simulink model "rgb2grey_hw"  (R2019a)
settings: Solver=FixedStepDiscrete  StartTime=0.0  StopTime=inf  RelTol=1e-3
undefined symbols (not defined in the file): HDTV, Rec
libraries: visionzynq_privlib x3, dspvision x1, hdlsllib x1, visionsinks x1, visionzynqlib x1
settings Model: DataTypeOverride=Off  SimulationMode=accelerator  Creator=lbai  LastModifiedBy=lbai
settings DataIOCC: LimitDataPoints=on  SaveOutput=off  SignalLogging=off  DSMLogging=off  VisualizeSimOutput=off  SaveTime=off
settings OptimizationCC: BlockReduction=off  ConditionallyExecuteInputs=off  DefaultParameterBehavior=Inlined  LifeSpan=inf  SimCompilerOptimization=on
settings DebuggingCC: AlgebraicLoopMsg=error  SingleTaskRateTransMsg=error  ParameterPrecisionLossMsg=none  AllowSymbolicDim=off  PregeneratedLibrarySubsystemCodeDiagnostic=none  SFUnexpectedBacktrackingDiag=warning  SFNoUnconditionalDefaultTransitionDiag=warning  SFExecutionAtInitializationDiag=none  IntegerSaturationMsg=none  ArithmeticOperatorsInVariantConditions=warning
settings HardwareCC: ProdBitPerPointer=32  ProdBitPerSizeT=32  ProdBitPerPtrDiffT=32  ProdLargestAtomicFloat=None  ProdIntDivRoundTo=Undefined  ProdEndianess=Unspecified  ProdWordSize=32  ProdHWDeviceType=ASIC/FPGA->ASIC/FPGA  ProdEqTarget=off
settings SFSimCC: SimUseLocalCustomCode=off
settings RTWCC: RTWUseLocalCustomCode=off  BuildConfiguration=Faster Runs
settings CodeAppCC: StateflowObjectComments=on
settings GRTTargetCC: TargetLangStandard=C89/C90 (ANSI)  GeneratePreprocessorConditionals=Disable all
settings ConfigComp: CovMetricSettings=dw  CovHtmlReporting=on  CovSaveCumulativeToWorkspaceVar=on  CovSaveSingleToWorkspaceVar=on  CovExternalEMLEnable=off  CovSFcnEnable=off

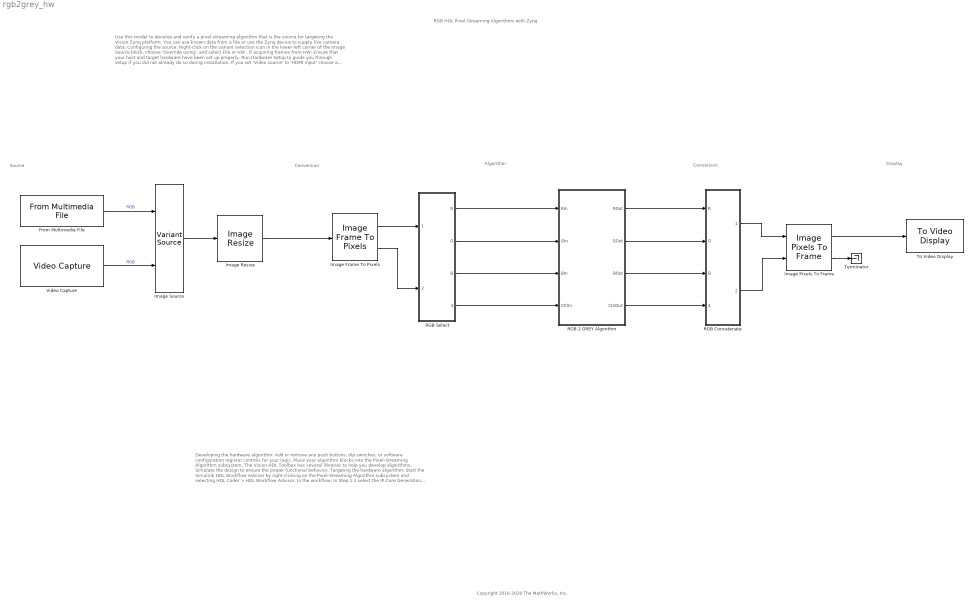
== system rgb2grey_hw ==
  note: Developing the hardware algorithm:
      | Add or remove any push buttons, dip switches, or software configuration register controls for your logic.
      | Place your algorithm blocks into the Pixel-Streaming Algorithm subsystem. The Vision HDL Toolbox has several libraries to help you develop algorithms.
      | Simulate the design to ensure the proper functional behavior.
      |
      | Targeting the hardware algorithm:
      |
      | Start the Simulink HDL Workflow Advisor by right-clicking on the Pixel-Streaming Algorithm subsystem and selecting HDL Coder > HDL Workflow Advisor.
      | In the workflow:
      | In Step 1.1 select the IP Core Generation workflow
      | In Step 1.1 select one of ZedBoard FMC-HDMI-CAM, ZC702 FMC-HDMI-CAM, ZC706 FMC-HDMI-CAM,
      | PicoZed FMC-HDMI-CAM.
      | In Step 1.2 select the reference platform that matches the desired pixel format.
      | In Step 1.3 map the reference design signals to the ports of the Pixel-Streaming Algorithm subsystem.
  note: Conversion
  note: Use this model to develop and verify a pixel-streaming algorithm that is the source for targeting the Vision Zynq platform. You can use known data from a file or use the Zynq device to supply live camera data.
      |
      | Configuring the source:
      | Right-click on the variant selection icon in the lower-left corner of the Image Source block, choose 'Override using', and select File or HW .
      | If acquiring frames from HW:
      | Ensure that your host and target hardware have been set up properly. Run Hardware Setup to guide you through setup if you did not already do so during installation.
      | If you set 'Video source' to 'HDMI input' choose a frame size that matches your camera settings.
      | If you set 'Video source' to 'Test pattern generator' choose any listed resolution. The hardware generates a color bar test pattern, and does not need an attached camera. It still requires the FMC board.
      | Since pixel-streaming algorithms will run many times slower than behavioral algorithms, consider adding a Resize block from Computer Vision System Toolbox to reduce the frame size that the algorithm operates on.
      |
      | Configuring conversions:
      | Ensure your Frame to Pixel and Pixel to Frame blocks match your source frame size.
  note: RGB HDL Pixel-Streaming Algorithms with Zynq
  note: Source
  note: Algorithm
  note: Display
  note: Conversion
  note: Copyright 2016-2018 The MathWorks, Inc.
  From Multimedia File : dspvision/From Multimedia File  inputFilename=vzSample1080p.avi  readRange=[1 Inf]  loop=on  numPlays=inf  outputStreams=Video only  videoDataType=uint8  audioDataType=int16  inheritSampleTime=off  userDefinedSampleTime=1/60  noAudioOutput=off  isIntensityVideo=off  fourcc=RGB  colorVideoFormat=One multidimensional signal  outputEOF=off  dataOrg=Column-major  audioFrameSize=1024  computeAudioFrameSize=off  outSamplingMode=Sample based
      settings: SourceProductName=DSP System Toolbox  SourceProductBaseCode=DS
  "Image Frame To Pixels " : visionzynq_privlib/Image Frame To Pixels   FrameSize=320x240p
      settings: SourceProductName=Computer Vision Toolbox Support Package for Xilinx Zynq-Based Hardware  SourceProductBaseCode=VP_VISION_ZYNQ
  Image Pixels To Frame : visionzynq_privlib/Image Pixels To Frame  FrameSize=320x240p
      settings: SourceProductName=Computer Vision Toolbox Support Package for Xilinx Zynq-Based Hardware  SourceProductBaseCode=VP_VISION_ZYNQ
  Image Resize : visionzynq_privlib/Image Resize  FrameSize=320x240p
      settings: SourceProductName=Computer Vision Toolbox Support Package for Xilinx Zynq-Based Hardware  SourceProductBaseCode=VP_VISION_ZYNQ
  Image Source : VariantSource  VariantControlMode=Label  LabelModeActiveChoice=File  ShowConditionOnBlock=on
  RGB 2 GREY Algorithm : Subsystem  TreatAsAtomicUnit=on
  RGB Concatenate : Subsystem
  RGB Select : Subsystem
  Terminator : Terminator
  To Video Display : visionsinks/To Video Display  windowSizeMode=Normal  openAtMdlStart=on  fullScreen=off  videoWindowX=536805376  videoWindowY=536805376  saveWindowSize=off  videoWindowWidth=2147483647  videoWindowHeight=2147483647  inputColorFormat=RGB  inputType=Obsolete  imagePorts=One multidimensional signal  OutputDevice=On-screen video monitor  dataOrg=Column-major  isWindowOpen=off
      settings: SourceProductName=Computer Vision Toolbox
  Video Capture : visionzynqlib/Video Capture  VideoSource=HDMI input  FrameSize=1080p HDTV (1920x1080p)  FrameRate=60fps  PixelFormatUI=RGB  CSCSpec=Rec. 709 (HDTV)  HWULBypass=off  CapturePoint=Input to FPGA user logic (A)  ROISource=No region of interest  ROIDimension=[100 100]  ROILocation=[1 1]  ImageSignal=One multidimensional signal  NoCameraHDMIMode=off  NoCameraHDMIColor=blue  CSCScanningStd=1125/60/2:1  TPGMode=Colorbars  TPGLevel=Line  TPGIncrement=bin2dec('0000')  EnablePixelFormat=on  MaskMode=Simulation
      settings: SourceProductName=Computer Vision Toolbox Support Package for Xilinx Zynq-Based Hardware  SourceProductBaseCode=VP_VISION_ZYNQ
  wires:
  "Image Frame To Pixels "/1 -> RGB Select/1(pixelData)
  "Image Frame To Pixels "/2 -> RGB Select/2(pixelCtrlIn)
  Image Pixels To Frame/2 -> Terminator/1
  Image Pixels To Frame/1 -> To Video Display/1
  RGB Concatenate/1(pixelData) -> Image Pixels To Frame/1
  RGB Concatenate/2(pixelCtrlOut) -> Image Pixels To Frame/2
  From Multimedia File/1 -> Image Source/1  "RGB"
  Video Capture/1 -> Image Source/2  "RGB"
  Image Source/1 -> Image Resize/1
  Image Resize/1 -> "Image Frame To Pixels "/1
  RGB Select/2(G) -> RGB 2 GREY Algorithm/2(GIn)
  RGB Select/1(R) -> RGB 2 GREY Algorithm/1(RIn)
  RGB Select/3(B) -> RGB 2 GREY Algorithm/3(BIn)
  RGB Select/4(pixelCtrlOut) -> RGB 2 GREY Algorithm/4(CtrlIn)
  RGB 2 GREY Algorithm/1(ROut) -> RGB Concatenate/1(R)
  RGB 2 GREY Algorithm/2(GOut) -> RGB Concatenate/2(G)
  RGB 2 GREY Algorithm/3(BOut) -> RGB Concatenate/3(B)
  RGB 2 GREY Algorithm/4(CtrlOut) -> RGB Concatenate/4(pixelCtrlIn)

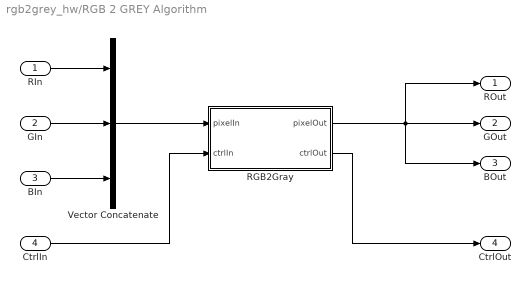
== system rgb2grey_hw/RGB 2 GREY Algorithm ==
  RIn : Inport
  GIn : Inport  Port=2
  BIn : Inport  Port=3
  CtrlIn : Inport  Port=4
  RGB2Gray : Subsystem
  Vector Concatenate : Concatenate  NumInputs=3  Mode=Multidimensional array  ConcatenateDimension=2
  ROut : Outport
  GOut : Outport  Port=2
  BOut : Outport  Port=3
  CtrlOut : Outport  Port=4
  wires:
  RIn/1 -> Vector Concatenate/1
  GIn/1 -> Vector Concatenate/2
  BIn/1 -> Vector Concatenate/3
  Vector Concatenate/1 -> RGB2Gray/1(pixelIn)
  CtrlIn/1 -> RGB2Gray/2(ctrlIn)
  RGB2Gray/2(ctrlOut) -> CtrlOut/1
  RGB2Gray/1(pixelOut) -> ROut/1, BOut/1, GOut/1

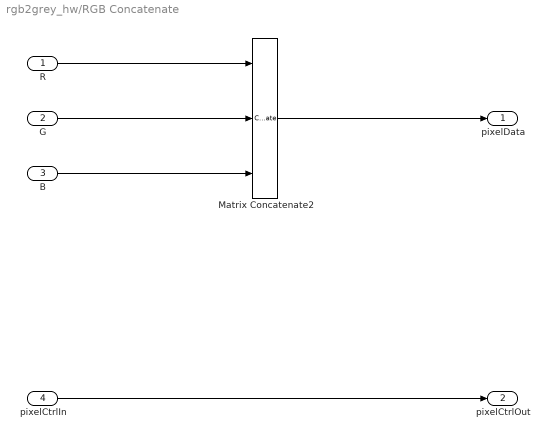
== system rgb2grey_hw/RGB Concatenate ==
  R : Inport
  G : Inport  Port=2
  B : Inport  Port=3
  pixelCtrlIn : Inport  Port=4
  Matrix Concatenate2 : Concatenate  NumInputs=3  Mode=Multidimensional array  ConcatenateDimension=2
  pixelData : Outport
  pixelCtrlOut : Outport  Port=2
  wires:
  R/1 -> Matrix Concatenate2/1
  G/1 -> Matrix Concatenate2/2
  Matrix Concatenate2/1 -> pixelData/1
  pixelCtrlIn/1 -> pixelCtrlOut/1
  B/1 -> Matrix Concatenate2/3

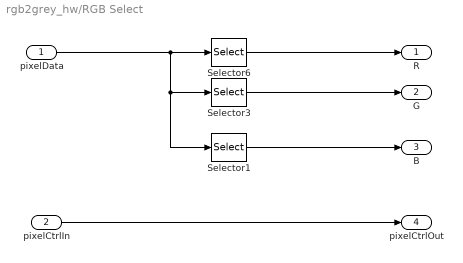
== system rgb2grey_hw/RGB Select ==
  pixelData : Inport
  pixelCtrlIn : Inport  Port=2
  Selector1 : Selector  NumberOfDimensions=2  InputPortWidth=3  IndexOptions=Select all,Index vector (dialog)  Indices=[1 3],3  OutputSizes=1,1
  Selector3 : Selector  NumberOfDimensions=2  InputPortWidth=3  IndexOptions=Select all,Index vector (dialog)  Indices=[1 3],2  OutputSizes=1,1
  Selector6 : Selector  NumberOfDimensions=2  InputPortWidth=3  IndexOptions=Select all,Index vector (dialog)  Indices=[1 3],1  OutputSizes=1,1
  R : Outport
  G : Outport  Port=2
  B : Outport  Port=3
  pixelCtrlOut : Outport  Port=4
  wires:
  pixelData/1 -> Selector1/1, Selector3/1, Selector6/1
  pixelCtrlIn/1 -> pixelCtrlOut/1
  Selector3/1 -> G/1
  Selector6/1 -> R/1
  Selector1/1 -> B/1

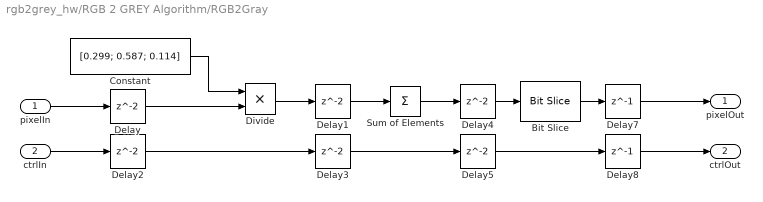
== system rgb2grey_hw/RGB 2 GREY Algorithm/RGB2Gray ==
  pixelIn : Inport
  ctrlIn : Inport  Port=2
  Bit Slice : hdlsllib/Logic and Bit Operations/Bit Slice  lidx=23  ridx=16
      settings: SourceProductName=Simulink  SourceProductBaseCode=SL
  Constant : Constant  Value=[0.299; 0.587; 0.114]  OutDataTypeStr=fixdt(0,16,16)  SampleTime=-1
  Delay{,1..5} (6 alike) : Delay
  Delay7 : Delay  DelayLength=1
  Delay8 : Delay  DelayLength=1
  Divide : Product  Inputs=**
  Sum of Elements : Sum  Inputs=+
  pixelOut : Outport  VectorParamsAs1DForOutWhenUnconnected=on
  ctrlOut : Outport  Port=2  VectorParamsAs1DForOutWhenUnconnected=on
  wires:
  Constant/1 -> Divide/1
  Divide/1 -> Delay1/1
  Delay5/1 -> Delay8/1
  Delay2/1 -> Delay3/1
  Bit Slice/1 -> Delay7/1
  Delay4/1 -> Bit Slice/1
  Delay/1 -> Divide/2
  Delay1/1 -> Sum of Elements/1
  Sum of Elements/1 -> Delay4/1
  Delay3/1 -> Delay5/1
  pixelIn/1 -> Delay/1
  Delay7/1 -> pixelOut/1
  ctrlIn/1 -> Delay2/1
  Delay8/1 -> ctrlOut/1
